simulink model "N_scheme_RP4"  (R2024b)
settings: Solver=VariableStepAuto  StartTime=0.0  StopTime=10.0  RelTol=1e-3
values from neighbouring files (symbols this model uses):
  Ga = -12500    [p23.m]
  Gf = 1/(Kd*Gs)    (= 0.25)    [p23.m]
  Gs = 2    [p23.m]
  K_n = (K_max+K_min)/2    (= 2)    [p23.m]
  p_n = (p_max+p_min)/2    (= 125)    [p23.m]
  Wk = (K_max-K_min)/2    (= 1)    [p23.m]
  Wp = (p_max-p_min)/2    (= 75)    [p23.m]
libraries: cstblocks x2
settings Model: Creator=adrian  LastModifiedBy=adrian

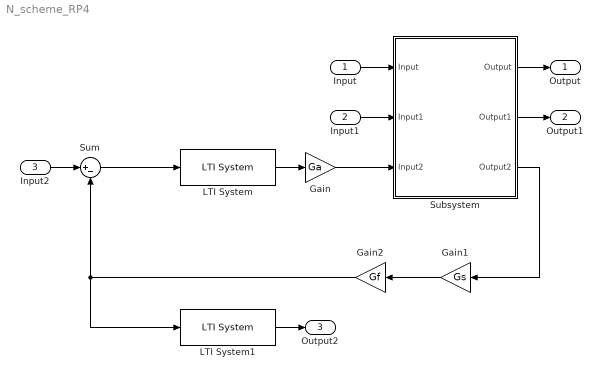
== system N_scheme_RP4 ==
  Input : Inport
  Input1 : Inport  Port=2
  Input2 : Inport  Port=3
  Gain : Gain  Gain=Ga
  Gain1 : Gain  Gain=Gs
  Gain2 : Gain  Gain=Gf
  LTI System : cstblocks/LTI System  sys=Gc  IC=[]  PadeOrder=0
  LTI System1 : cstblocks/LTI System  sys=WT_mu_RP4  IC=[]  PadeOrder=0
  Subsystem : Subsystem
  Sum : Sum  Inputs=|+-
  Output : Outport
  Output1 : Outport  Port=2
  Output2 : Outport  Port=3
  wires:
  Gain/1 -> Subsystem/3(Input2)
  Input/1 -> Subsystem/1(Input)
  Input1/1 -> Subsystem/2(Input1)
  LTI System/1 -> Gain/1
  Subsystem/3(Output2) -> Gain1/1
  Subsystem/1(Output) -> Output/1
  Subsystem/2(Output1) -> Output1/1
  Gain1/1 -> Gain2/1
  Gain2/1 -> Sum/2, LTI System1/1
  Sum/1 -> LTI System/1
  Input2/1 -> Sum/1
  LTI System1/1 -> Output2/1

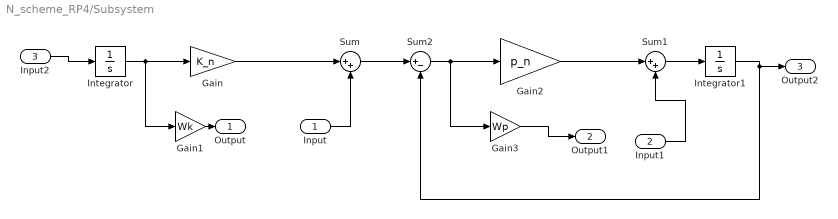
== system N_scheme_RP4/Subsystem ==
  Input : Inport
  Input1 : Inport  Port=2
  Input2 : Inport  Port=3
  Gain : Gain  Gain=K_n
  Gain1 : Gain  Gain=Wk
  Gain2 : Gain  Gain=p_n
  Gain3 : Gain  Gain=Wp
  Integrator : Integrator
  Integrator1 : Integrator
  Sum : Sum  Inputs=|++
  Sum1 : Sum  Inputs=|++
  Sum2 : Sum  Inputs=|+-
  Output : Outport
  Output1 : Outport  Port=2
  Output2 : Outport  Port=3
  wires:
  Integrator/1 -> Gain1/1, Gain/1
  Gain/1 -> Sum/1
  Gain1/1 -> Output/1
  Input/1 -> Sum/2
  Sum2/1 -> Gain3/1, Gain2/1
  Sum/1 -> Sum2/1
  Sum1/1 -> Integrator1/1
  Gain2/1 -> Sum1/1
  Integrator1/1 -> Output2/1, Sum2/2
  Input1/1 -> Sum1/2
  Gain3/1 -> Output1/1
  Input2/1 -> Integrator/1
